simulink model "orientation"  (R2017b)
settings: Solver=ode4  StartTime=0.0  StopTime=1  FixedStep=0.01  RelTol=1e-3
settings Model: Creator=wol4aravio  LastModifiedBy=wol4aravio
settings DataIOCC: ExternalInput=[a, b]  SaveOutput=off  SignalLogging=off  DSMLogging=off  SaveTime=off

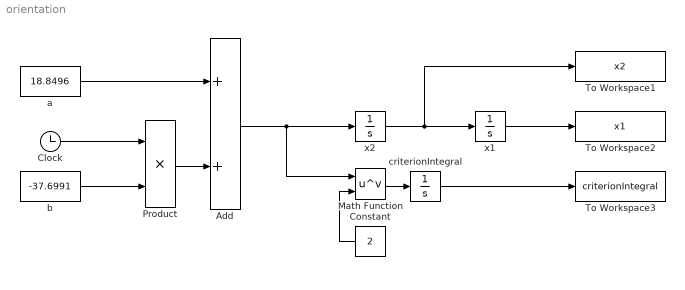
== system orientation ==
  Add : Sum
  Clock : Clock
  Constant : Constant  Value=2
  Math Function : Math  Operator=pow  SaturateOnIntegerOverflow=on
  Product : Product
  To Workspace1 : ToWorkspace  VariableName=x2  SaveFormat=Timeseries  SampleTime=-1
  To Workspace2 : ToWorkspace  VariableName=x1  SaveFormat=Timeseries  SampleTime=-1
  To Workspace3 : ToWorkspace  VariableName=criterionIntegral  SaveFormat=Timeseries  SampleTime=-1
  a : Constant  Value=18.8496
  b : Constant  Value=-37.6991
  criterionIntegral : Integrator  ContinuousStateAttributes='criterionIntegral'
  x1 : Integrator  ContinuousStateAttributes='x1'
  x2 : Integrator  ContinuousStateAttributes='x2'
  wires:
  Clock/1 -> Product/1
  b/1 -> Product/2
  Product/1 -> Add/2
  a/1 -> Add/1
  Add/1 -> Math Function/1, x2/1
  x2/1 -> To Workspace1/1, x1/1
  Math Function/1 -> criterionIntegral/1
  Constant/1 -> Math Function/2
  criterionIntegral/1 -> To Workspace3/1
  x1/1 -> To Workspace2/1
